simulink model "Prova_SITL_GPS_2020b"  (R2020b)
settings: Solver=VariableStepAuto  StartTime=0.0  StopTime=10  RelTol=1e-3
values from neighbouring files (symbols this model uses):
  K = 0.5*rho*v^2*S*cbar    (= 36.62030592)    [v2021_10_27_calcoloAerodinamica.m]
  sw = 5    [Dati_prova_GPS_SITL.m]    (also in modellazione_erroe_GPS.m = input('inserire simulazione richiesta '))
libraries: simulink x3
settings Model: Creator=User  LastModifiedBy=User

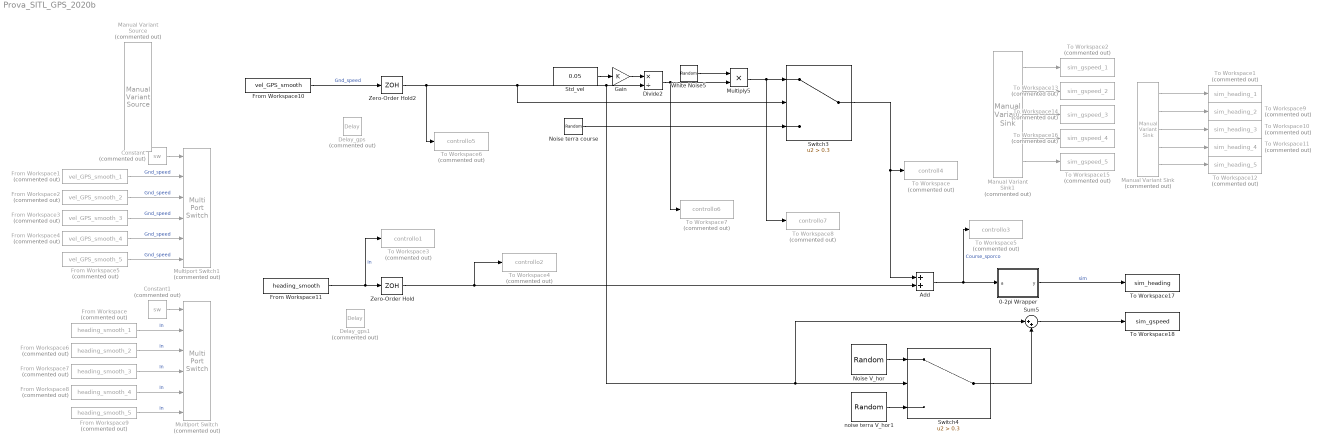
== system Prova_SITL_GPS_2020b ==
  0-2pi Wrapper : MATLAB Function  TreatAsAtomicUnit=on
  Add : Sum
  Constant : Constant  Commented=on  Value=sw
  Constant1 : Constant  Commented=on  Value=sw
  Delay_gps : TransportDelay  Commented=on  DelayTime=0
  Delay_gps1 : TransportDelay  Commented=on  DelayTime=0
  Divide2 : Product  Inputs=*/
  From Workspace : FromWorkspace  Commented=on  VariableName=heading_smooth_1
  From Workspace1 : FromWorkspace  Commented=on  VariableName=vel_GPS_smooth_1
  From Workspace10 : FromWorkspace  VariableName=vel_GPS_smooth
  From Workspace11 : FromWorkspace  VariableName=heading_smooth
  From Workspace2 : FromWorkspace  Commented=on  VariableName=vel_GPS_smooth_2
  From Workspace3 : FromWorkspace  Commented=on  VariableName=vel_GPS_smooth_3
  From Workspace4 : FromWorkspace  Commented=on  VariableName=vel_GPS_smooth_4
  From Workspace5 : FromWorkspace  Commented=on  VariableName=vel_GPS_smooth_5
  From Workspace6 : FromWorkspace  Commented=on  VariableName=heading_smooth_2
  From Workspace7 : FromWorkspace  Commented=on  VariableName=heading_smooth_3
  From Workspace8 : FromWorkspace  Commented=on  VariableName=heading_smooth_4
  From Workspace9 : FromWorkspace  Commented=on  VariableName=heading_smooth_5
  Gain : Gain  Gain=K
  Manual Variant Sink : simulink/Signal Routing/Manual Variant Sink  Commented=on  NumChoices=5  LabelModeActiveChoice=V_1
  Manual Variant Sink1 : simulink/Signal Routing/Manual Variant Sink  Commented=on  NumChoices=5  LabelModeActiveChoice=V_1
  Manual Variant Source : simulink/Signal Routing/Manual Variant Source  Commented=on  NumChoices=5  LabelModeActiveChoice=V_1
  Multiply5 : Product
  Multiport Switch : MultiPortSwitch  Commented=on  DataPortOrder=Specify indices  Inputs=5  DataPortIndices={1,2,3,4,5}
  Multiport Switch1 : MultiPortSwitch  Commented=on  DataPortOrder=Specify indices  Inputs=5  DataPortIndices={1,2,3,4,5}
  Noise V_hor : RandomNumber  Variance=0.025  Seed=randi([0 2000],1,1)  SampleTime=0.2
  Noise terra course : RandomNumber  Variance=0.2  Seed=randi([0 2000],1,1)  SampleTime=0.02
  Std_vel : Constant  Value=0.05
  Sum5 : Sum  Inputs=|++
  Switch3 : Switch  Criteria=u2 > Threshold  Threshold=0.3
  Switch4 : Switch  Criteria=u2 > Threshold  Threshold=0.3
  To Workspace : ToWorkspace  Commented=on  VariableName=controll4  SampleTime=-1
  To Workspace1 : ToWorkspace  Commented=on  VariableName=sim_heading_1  SampleTime=-1
      settings: Save2DSignal=2-D array (concatenate along first dimension)
  To Workspace10 : ToWorkspace  Commented=on  VariableName=sim_heading_3  SampleTime=-1
      settings: Save2DSignal=2-D array (concatenate along first dimension)
  To Workspace11 : ToWorkspace  Commented=on  VariableName=sim_heading_4  SampleTime=-1
      settings: Save2DSignal=2-D array (concatenate along first dimension)
  To Workspace12 : ToWorkspace  Commented=on  VariableName=sim_heading_5  SampleTime=-1
      settings: Save2DSignal=2-D array (concatenate along first dimension)
  To Workspace13 : ToWorkspace  Commented=on  VariableName=sim_gspeed_2  SampleTime=-1
      settings: Save2DSignal=2-D array (concatenate along first dimension)
  To Workspace14 : ToWorkspace  Commented=on  VariableName=sim_gspeed_3  SampleTime=-1
      settings: Save2DSignal=2-D array (concatenate along first dimension)
  To Workspace15 : ToWorkspace  Commented=on  VariableName=sim_gspeed_5  SampleTime=-1
      settings: Save2DSignal=2-D array (concatenate along first dimension)
  To Workspace16 : ToWorkspace  Commented=on  VariableName=sim_gspeed_4  SampleTime=-1
      settings: Save2DSignal=2-D array (concatenate along first dimension)
  To Workspace17 : ToWorkspace  VariableName=sim_heading  SampleTime=-1
  To Workspace18 : ToWorkspace  VariableName=sim_gspeed  SampleTime=-1
  To Workspace2 : ToWorkspace  Commented=on  VariableName=sim_gspeed_1  SampleTime=-1
      settings: Save2DSignal=2-D array (concatenate along first dimension)
  To Workspace3 : ToWorkspace  Commented=on  VariableName=controllo1  SampleTime=-1
      settings: Save2DSignal=2-D array (concatenate along first dimension)
  To Workspace4 : ToWorkspace  Commented=on  VariableName=controllo2  SampleTime=-1
      settings: Save2DSignal=2-D array (concatenate along first dimension)
  To Workspace5 : ToWorkspace  Commented=on  VariableName=controllo3  SampleTime=-1
      settings: Save2DSignal=2-D array (concatenate along first dimension)
  To Workspace6 : ToWorkspace  Commented=on  VariableName=controllo5  SampleTime=-1
      settings: Save2DSignal=2-D array (concatenate along first dimension)
  To Workspace7 : ToWorkspace  Commented=on  VariableName=controllo6  SampleTime=-1
      settings: Save2DSignal=2-D array (concatenate along first dimension)
  To Workspace8 : ToWorkspace  Commented=on  VariableName=controllo7  SampleTime=-1
      settings: Save2DSignal=2-D array (concatenate along first dimension)
  To Workspace9 : ToWorkspace  Commented=on  VariableName=sim_heading_2  SampleTime=-1
      settings: Save2DSignal=2-D array (concatenate along first dimension)
  White Noise5 : RandomNumber  Variance=0.1  Seed=randi([0 2000],1,1)  SampleTime=0.02
  Zero-Order Hold : ZeroOrderHold  SampleTime=0.02
  Zero-Order Hold2 : ZeroOrderHold  SampleTime=0.02
  noise terra V_hor1 : RandomNumber  Variance=0.25  Seed=randi([0 2000],1,1)  SampleTime=0.2
  wires:
  Std_vel/1 -> Gain/1
  From Workspace11/1 -> To Workspace3/1, Zero-Order Hold/1  "In"
  Switch4/1 -> Sum5/2
  Add/1 -> To Workspace5/1, 0-2pi Wrapper/1(a)  "Course_sporco"
  noise terra V_hor1/1 -> Switch4/3
  Zero-Order Hold2/1 -> To Workspace6/1, Switch3/2, Divide2/2, Switch4/2, Sum5/1
  Gain/1 -> Divide2/1
  From Workspace10/1 -> Zero-Order Hold2/1  "Gnd_speed"
  Noise terra course/1 -> Switch3/3
  Switch3/1 -> To Workspace/1, Add/1
  Noise V_hor/1 -> Switch4/1
  White Noise5/1 -> Multiply5/1
  0-2pi Wrapper/1(y) -> To Workspace17/1  "sim"
  Sum5/1 -> To Workspace18/1
  Zero-Order Hold/1 -> To Workspace4/1, Add/2
  Divide2/1 -> To Workspace7/1, Multiply5/2
  Multiply5/1 -> To Workspace8/1, Switch3/1
  From Workspace/1 -> Multiport Switch/2  "In"
  From Workspace1/1 -> Multiport Switch1/2  "Gnd_speed"
  From Workspace2/1 -> Multiport Switch1/3  "Gnd_speed"
  From Workspace3/1 -> Multiport Switch1/4  "Gnd_speed"
  From Workspace4/1 -> Multiport Switch1/5  "Gnd_speed"
  From Workspace5/1 -> Multiport Switch1/6  "Gnd_speed"
  From Workspace6/1 -> Multiport Switch/3  "In"
  From Workspace7/1 -> Multiport Switch/4  "In"
  From Workspace8/1 -> Multiport Switch/5  "In"
  From Workspace9/1 -> Multiport Switch/6  "In"
  Manual Variant Sink/1 -> To Workspace1/1
  Manual Variant Sink/2 -> To Workspace9/1
  Manual Variant Sink/3 -> To Workspace10/1
  Manual Variant Sink/4 -> To Workspace11/1
  Manual Variant Sink/5 -> To Workspace12/1
  Manual Variant Sink1/1 -> To Workspace2/1
  Manual Variant Sink1/2 -> To Workspace13/1
  Manual Variant Sink1/3 -> To Workspace14/1
  Manual Variant Sink1/5 -> To Workspace15/1
  Manual Variant Sink1/4 -> To Workspace16/1
  Constant/1 -> Multiport Switch1/1
  Constant1/1 -> Multiport Switch/1

== matlab function Prova_SITL_GPS_2020b/0-2pi Wrapper ==
  data: a input; y output
function y = fcn(a)
%% Wrapper da [-180,+180] a [0,360]
%https://stackoverflow.com/questions/11498169/dealing-with-angle-wrap-in-c-code
close all

b=2*pi;

k=floor(a/b);
fmod=a-k*b;


if fmod<0
    
   fmod=fmod+2*pi;
    
end

y=fmod;
